simulink model "deltasigma1"  (Simulink 7.6)
settings: Solver=ode45  StartTime=0  StopTime=1  RelTol=1e-3
libraries: simeventssignalmanage1 x3, dsparch4 x1, simulink_extras x1, simulink x1
settings Model: Creator=Robin  LastModifiedBy=Robin
settings DebuggingCC: SolverPrmCheckMsg=none
settings SimEventsCC: propDiagAttribOutput=1  propDiagFcnCallOutput=1  propDiagStatOutput=0

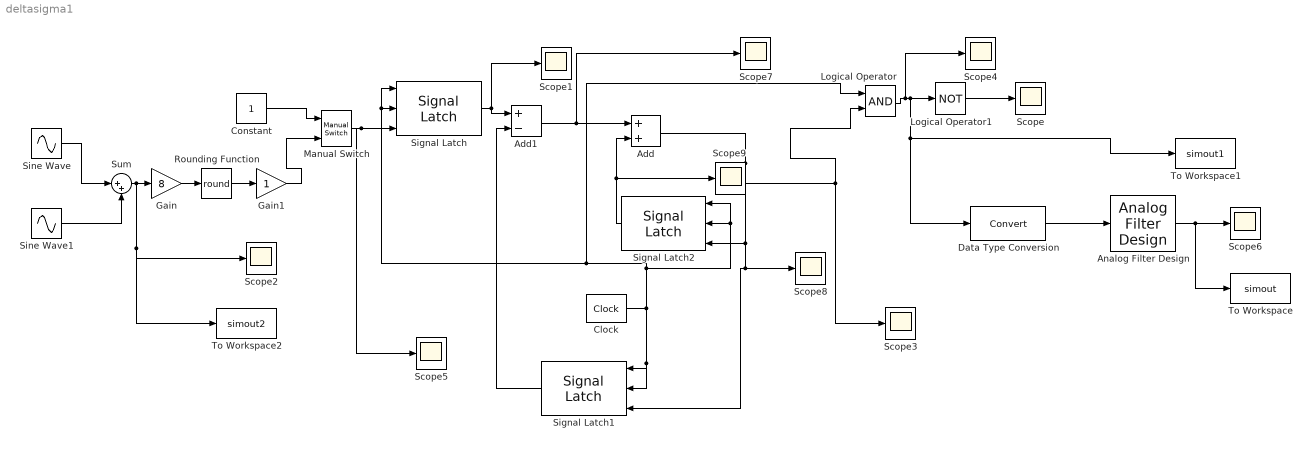
== system deltasigma1 ==
  Add : Sum  AccumDataTypeStr=int16  RndMeth=Convergent
  Add1 : Sum  Inputs=+-  AccumDataTypeStr=int16  RndMeth=Convergent
  Analog Filter Design : dsparch4/Analog Filter Design  method=Butterworth  filttype=Lowpass  N=2  Wlo=30*pi  Whi=10*pi  Rp=2  Rs=40
  Clock : simulink_extras/Flip Flops/Clock  SystemSampleTime=-1  period=1/400
  Constant : Constant
  Data Type Conversion : DataTypeConversion  RndMeth=Convergent
  Gain : Gain  Gain=8
  Gain1 : Gain
  Logical Operator : Logic  AllPortsSameDT=off
  Logical Operator1 : Logic  Operator=NOT  AllPortsSameDT=off  OutDataTypeStr=boolean
  Manual Switch : simulink/Signal Routing/Manual Switch  SystemSampleTime=-1  sw=0  action=0  varsize=off
  Rounding Function : Rounding  Operator=round
  Scope{,1..9} (10 alike) : Scope
      Scope2 settings: SaveName=ScopeData2
      Scope3 settings: TimeRange=10  YMin=-1  YMax=2  SaveName=ScopeData3
      Scope4 settings: SaveName=ScopeData4
      Scope5 settings: SaveName=ScopeData5
      Scope6 settings: YMin=-1  YMax=1  SaveName=ScopeData6
      Scope7 settings: SaveName=ScopeData7
      Scope8 settings: SaveName=ScopeData8
      Scope9 settings: SaveName=ScopeData9
  Signal Latch : simeventssignalmanage1/Signal Latch  SystemSampleTime=-1  InitialMemoryValue=0  WriteMemoryUpon=Change in signal from port wvc  MemoryWriteEdgeOption=Rising  SpecifyWriteEventPriority=on  PriorityMemoryWrite=7100  ReadMemoryUpon=Change in signal from port rvc  MemoryReadEdgeOption=Falling  SpecifyReadEventPriority=on  PriorityMemoryRead=7000  ReportMemoryState=off  ReportMemoryUponWrite=off  ReportMemoryUponRead=on
  Signal Latch1 : simeventssignalmanage1/Signal Latch  SystemSampleTime=-1  InitialMemoryValue=0  WriteMemoryUpon=Change in signal from port wvc  MemoryWriteEdgeOption=Rising  SpecifyWriteEventPriority=on  PriorityMemoryWrite=7100  ReadMemoryUpon=Change in signal from port rvc  MemoryReadEdgeOption=Falling  SpecifyReadEventPriority=on  PriorityMemoryRead=7000  ReportMemoryState=off  ReportMemoryUponWrite=off  ReportMemoryUponRead=on
  Signal Latch2 : simeventssignalmanage1/Signal Latch  SystemSampleTime=-1  InitialMemoryValue=0  WriteMemoryUpon=Change in signal from port wvc  MemoryWriteEdgeOption=Rising  SpecifyWriteEventPriority=on  PriorityMemoryWrite=7100  ReadMemoryUpon=Change in signal from port rvc  MemoryReadEdgeOption=Falling  SpecifyReadEventPriority=on  PriorityMemoryRead=7000  ReportMemoryState=off  ReportMemoryUponWrite=off  ReportMemoryUponRead=on
  Sine Wave : Sin  Bias=1  Frequency=20*pi  SampleTime=0
  Sine Wave1 : Sin  Frequency=40*pi  SampleTime=0
  Sum : Sum  Inputs=|++
  To Workspace : ToWorkspace  VariableName=simout  SampleTime=-1  SaveFormat=Structure With Time
  To Workspace1 : ToWorkspace  VariableName=simout1  SampleTime=-1  SaveFormat=Structure With Time
  To Workspace2 : ToWorkspace  VariableName=simout2  SampleTime=-1  SaveFormat=Structure With Time
  wires:
  Add1/1 -> Add/1, Scope7/1
  Signal Latch/1 -> Scope1/1, Add1/1
  Signal Latch2/1 -> Add/2, Scope9/1
  Logical Operator/1 -> Scope4/1, Logical Operator1/1, Data Type Conversion/1, To Workspace1/1
  Clock/1 -> Signal Latch2/1, Signal Latch2/2, Signal Latch/1, Signal Latch/2, Logical Operator/1, Signal Latch1/1, Signal Latch1/2
  Logical Operator1/1 -> Scope/1
  Add/1 -> Signal Latch2/3, Scope8/1, Signal Latch1/3, Logical Operator/2, Scope3/1
  Analog Filter Design/1 -> Scope6/1, To Workspace/1
  Data Type Conversion/1 -> Analog Filter Design/1
  Gain1/1 -> Manual Switch/2
  Constant/1 -> Manual Switch/1
  Gain/1 -> Rounding Function/1
  Rounding Function/1 -> Gain1/1
  Sine Wave1/1 -> Sum/2
  Sum/1 -> Gain/1, To Workspace2/1, Scope2/1
  Signal Latch1/1 -> Add1/2
  Sine Wave/1 -> Sum/1
  Manual Switch/1 -> Signal Latch/3, Scope5/1
